simulink model "testfuzzy"  (R2018b)
settings: Solver=ode15s  StartTime=0.0  StopTime=10.0  MaxStep=0.1  RelTol=1e-3
values from neighbouring files (symbols this model uses):
  F = [         1, 2, 3, 1;         1, 3, 4, 1;         1, 2, 5, 1;         1, 5, 4, 1;         2, 3, 6, 2;         3, 4, 6, 3;         2, 5, 6, 2;         4, 5, 6, 4;         6, 15, 16, 6;         7, 8, 9, 10;         11, 12, 13, 14;         ]    [drawVehicle.m]    (also in draw_runway.m)
  q = uu(11)    [drawVehicle.m]    (also in forceee.m; plotmavstatevariables.m = 180/pi*uu(11); plotresults.m = 180/pi*uu(11))
  r = uu(12)    [drawVehicle.m]    (also in forceee.m; plotmavstatevariables.m = 180/pi*uu(12); plotresults.m = 180/pi*uu(12))
undefined symbols (not defined in the file or in its folder): altitude_state_machine, drawVehicle, forceee, forces_moments, gps, Light, MIL, P, plotmavstatevariables, plotresults, sensors, true_states
libraries: simulink_extras x9, fuzblock x8, aerolibwind2 x4, sharedtransform x2, simulink x2, aerolibobsolete x1
(part 2 of 2)

== system testfuzzy/Autopilot/Pitch Command Control/Airspeed Hold Using Pitch Loop PI Control /Altitude State Check ==
  err_in : Inport
  Descend Zone : Constant  Value=4
  Product : Product
  Relational Operator : RelationalOperator  Operator===  OutDataTypeStr=boolean  RndMeth=Simplest
  err_out : Outport
  wires:
  err_in/1 -> Product/2
  Relational Operator/1 -> Product/1
  Product/1 -> err_out/1
  [alt_state] -> Relational Operator/1
  Descend Zone/1 -> Relational Operator/2

== system testfuzzy/Autopilot/Pitch Command Control/Altitude Hold Using Pitch Loop PI Control/Altitude State Check ==
  err_in : Inport
  Alt Hold Zone : Constant  Value=3
  Product : Product
  Relational Operator : RelationalOperator  Operator===  OutDataTypeStr=boolean  RndMeth=Simplest
  err_out : Outport
  wires:
  err_in/1 -> Product/2
  Relational Operator/1 -> Product/1
  Product/1 -> err_out/1
  [alt_state] -> Relational Operator/1
  Alt Hold Zone/1 -> Relational Operator/2

== system testfuzzy/Autopilot/Pitch Command Control1/Airspeed Hold Using Pitch Loop PI Control/Altitude State Check ==
  err_in : Inport
  Climb Zone : Constant  Value=2
  Product : Product
  Relational Operator : RelationalOperator  Operator===  OutDataTypeStr=boolean  RndMeth=Simplest
  err_out : Outport
  wires:
  err_in/1 -> Product/2
  Relational Operator/1 -> Product/1
  Product/1 -> err_out/1
  [alt_state] -> Relational Operator/1
  Climb Zone/1 -> Relational Operator/2

== system testfuzzy/Autopilot/Pitch Command Control1/Airspeed Hold Using Pitch Loop PI Control /Altitude State Check ==
  err_in : Inport
  Descend Zone : Constant  Value=4
  Product : Product
  Relational Operator : RelationalOperator  Operator===  OutDataTypeStr=boolean  RndMeth=Simplest
  err_out : Outport
  wires:
  err_in/1 -> Product/2
  Relational Operator/1 -> Product/1
  Product/1 -> err_out/1
  [alt_state] -> Relational Operator/1
  Descend Zone/1 -> Relational Operator/2

== system testfuzzy/Autopilot/Pitch Command Control1/Altitude Hold Using Pitch Loop PI Control/Altitude State Check ==
  err_in : Inport
  Alt Hold Zone : Constant  Value=3
  Product : Product
  Relational Operator : RelationalOperator  Operator===  OutDataTypeStr=boolean  RndMeth=Simplest
  err_out : Outport
  wires:
  err_in/1 -> Product/2
  Relational Operator/1 -> Product/1
  Product/1 -> err_out/1
  [alt_state] -> Relational Operator/1
  Alt Hold Zone/1 -> Relational Operator/2

== system testfuzzy/Autopilot/Pitch Command Control2/Airspeed Hold Using Pitch Loop PI Control/Altitude State Check ==
  err_in : Inport
  Climb Zone : Constant  Value=2
  Product : Product
  Relational Operator : RelationalOperator  Operator===  OutDataTypeStr=boolean  RndMeth=Simplest
  err_out : Outport
  wires:
  err_in/1 -> Product/2
  Relational Operator/1 -> Product/1
  Product/1 -> err_out/1
  [alt_state] -> Relational Operator/1
  Climb Zone/1 -> Relational Operator/2

== system testfuzzy/Autopilot/Pitch Command Control2/Airspeed Hold Using Pitch Loop PI Control /Altitude State Check ==
  err_in : Inport
  Descend Zone : Constant  Value=4
  Product : Product
  Relational Operator : RelationalOperator  Operator===  OutDataTypeStr=boolean  RndMeth=Simplest
  err_out : Outport
  wires:
  err_in/1 -> Product/2
  Relational Operator/1 -> Product/1
  Product/1 -> err_out/1
  [alt_state] -> Relational Operator/1
  Descend Zone/1 -> Relational Operator/2

== system testfuzzy/Autopilot/Pitch Command Control2/Altitude Hold Using Pitch Loop PI Control/Altitude State Check ==
  err_in : Inport
  Alt Hold Zone : Constant  Value=3
  Product : Product
  Relational Operator : RelationalOperator  Operator===  OutDataTypeStr=boolean  RndMeth=Simplest
  err_out : Outport
  wires:
  err_in/1 -> Product/2
  Relational Operator/1 -> Product/1
  Product/1 -> err_out/1
  [alt_state] -> Relational Operator/1
  Alt Hold Zone/1 -> Relational Operator/2

== system testfuzzy/Autopilot/Pitch Command Control3/Airspeed Hold Using Pitch Loop PI Control/Altitude State Check ==
  err_in : Inport
  Climb Zone : Constant  Value=2
  Product : Product
  Relational Operator : RelationalOperator  Operator===  OutDataTypeStr=boolean  RndMeth=Simplest
  err_out : Outport
  wires:
  err_in/1 -> Product/2
  Relational Operator/1 -> Product/1
  Product/1 -> err_out/1
  [alt_state] -> Relational Operator/1
  Climb Zone/1 -> Relational Operator/2

== system testfuzzy/Autopilot/Pitch Command Control3/Airspeed Hold Using Pitch Loop PI Control /Altitude State Check ==
  err_in : Inport
  Descend Zone : Constant  Value=4
  Product : Product
  Relational Operator : RelationalOperator  Operator===  OutDataTypeStr=boolean  RndMeth=Simplest
  err_out : Outport
  wires:
  err_in/1 -> Product/2
  Relational Operator/1 -> Product/1
  Product/1 -> err_out/1
  [alt_state] -> Relational Operator/1
  Descend Zone/1 -> Relational Operator/2

== system testfuzzy/Autopilot/Pitch Command Control3/Altitude Hold Using Pitch Loop PI Control/Altitude State Check ==
  err_in : Inport
  Alt Hold Zone : Constant  Value=3
  Product : Product
  Relational Operator : RelationalOperator  Operator===  OutDataTypeStr=boolean  RndMeth=Simplest
  err_out : Outport
  wires:
  err_in/1 -> Product/2
  Relational Operator/1 -> Product/1
  Product/1 -> err_out/1
  [alt_state] -> Relational Operator/1
  Alt Hold Zone/1 -> Relational Operator/2

== system testfuzzy/Autopilot/Throttle Control/Airspeed Hold Using Throttle PI Control/Altitude State Check ==
  err_in : Inport
  Alt Hold Zone : Constant  Value=3
  Product : Product
  Relational Operator : RelationalOperator  Operator===  OutDataTypeStr=boolean  RndMeth=Simplest
  err_out : Outport
  wires:
  err_in/1 -> Product/2
  Relational Operator/1 -> Product/1
  Product/1 -> err_out/1
  [alt_state] -> Relational Operator/1
  Alt Hold Zone/1 -> Relational Operator/2

== system testfuzzy/Autopilot/Throttle Control/Airspeed Hold Using Throttle PI Control1/Altitude State Check ==
  err_in : Inport
  Alt Hold Zone : Constant  Value=3
  Product : Product
  Relational Operator : RelationalOperator  Operator===  OutDataTypeStr=boolean  RndMeth=Simplest
  err_out : Outport
  wires:
  err_in/1 -> Product/2
  Relational Operator/1 -> Product/1
  Product/1 -> err_out/1
  [alt_state] -> Relational Operator/1
  Alt Hold Zone/1 -> Relational Operator/2
